simulink model "Kaltitude"  (R2015a)
settings: Solver=ode2  StartTime=0.0  StopTime=10.0  FixedStep=0.01  RelTol=1e-3
InitFcn:
  | Parameters
settings Model: Creator=pela  LastModifiedBy=Mattia
settings HardwareCC: ProdLargestAtomicInteger=Long  ProdLargestAtomicFloat=Double  ProdEndianess=LittleEndian  ProdHWDeviceType=ARM Compatible->ARM Cortex
settings RTWCC: GenCodeOnly=on  GenerateReport=on  Toolchain=Microsoft Visual C++ 2013 v12.0 | nmake (64-bit Windows)  BuildConfiguration=Faster Runs  LaunchReport=on  TargetLang=C++
settings GRTTargetCC: MatFileLogging=off  MultiInstanceERTCode=on  CodeInterfacePackaging=C++ class  SupportNonFinite=off

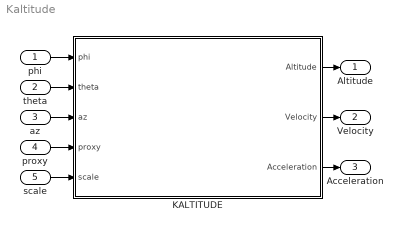
== system Kaltitude ==
  phi : Inport
  theta : Inport  Port=2
  az : Inport  Port=3
  proxy : Inport  Port=4
  scale : Inport  Port=5
  KALTITUDE : Subsystem
  Altitude : Outport
  Velocity : Outport  Port=2
  Acceleration : Outport  Port=3
  wires:
  phi/1 -> KALTITUDE/1(phi)
  theta/1 -> KALTITUDE/2(theta)
  az/1 -> KALTITUDE/3(az)
  proxy/1 -> KALTITUDE/4(proxy)
  KALTITUDE/1(Altitude) -> Altitude/1
  KALTITUDE/2(Velocity) -> Velocity/1
  KALTITUDE/3(Acceleration) -> Acceleration/1
  scale/1 -> KALTITUDE/5(scale)

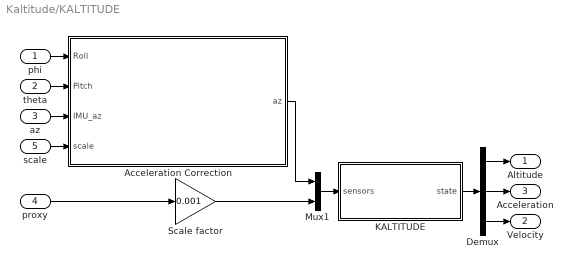
== system Kaltitude/KALTITUDE ==
  phi : Inport
  theta : Inport  Port=2
  az : Inport  Port=3
  proxy : Inport  Port=4
  scale : Inport  Port=5
  Acceleration Correction : MATLAB Function  TreatAsAtomicUnit=on
  Demux : Demux  Outputs=3
  KALTITUDE : Subsystem
  Mux1 : Mux  Inputs=2
  Scale factor : Gain  Gain=0.001
  Altitude : Outport
  Velocity : Outport  Port=2
  Acceleration : Outport  Port=3
  wires:
  az/1 -> Acceleration Correction/3(IMU_az)
  phi/1 -> Acceleration Correction/1(Roll)
  theta/1 -> Acceleration Correction/2(Pitch)
  Mux1/1 -> KALTITUDE/1(sensors)
  proxy/1 -> Scale factor/1
  Scale factor/1 -> Mux1/2
  Acceleration Correction/1(az) -> Mux1/1
  KALTITUDE/1(state) -> Demux/1
  Demux/1 -> Altitude/1
  Demux/2 -> Acceleration/1
  Demux/3 -> Velocity/1
  scale/1 -> Acceleration Correction/4(scale)

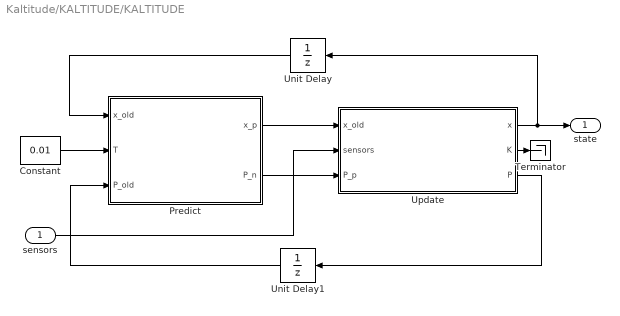
== system Kaltitude/KALTITUDE/KALTITUDE ==
  sensors : Inport
  Constant : Constant  Value=0.01  VectorParams1D=off  SampleTime=-1
  "Predict " : MATLAB Function  TreatAsAtomicUnit=on
  Terminator : Terminator
  Unit Delay : UnitDelay  InitialCondition=zeros(3,1)  SampleTime=-1
  Unit Delay1 : UnitDelay  InitialCondition=eye(3)*0.001  SampleTime=-1
  Update : MATLAB Function  TreatAsAtomicUnit=on
  state : Outport
  wires:
  Update/2(K) -> Terminator/1
  Unit Delay1/1 -> "Predict "/3(P_old)
  Update/1(x) -> state/1, Unit Delay/1
  "Predict "/1(x_p) -> Update/1(x_old)
  sensors/1 -> Update/2(sensors)
  "Predict "/2(P_n) -> Update/3(P_p)
  Constant/1 -> "Predict "/2(T)
  Update/3(P) -> Unit Delay1/1
  Unit Delay/1 -> "Predict "/1(x_old)

== matlab function Kaltitude/KALTITUDE/Acceleration Correction ==
  data: Roll input; Pitch input; IMU_az input; scale input; az output
function az = Accelerometer_correction(Roll,Pitch,IMU_az,scale)
%#codegen
acc_norm = IMU_az/scale;
a_corr = sqrt(1 - (sin(Roll)^2 + sin(Pitch)^2));

az = (acc_norm - a_corr)*9.81;

== matlab function Kaltitude/KALTITUDE/KALTITUDE/Update ==
  data x_old settings: description=A-priori state estimate.
  data sensors settings: description=Measurements from the sensors.
  data x settings: description=Corrected state estimate.
  data P_p settings: description=A-priori covariance estimate.
  data P settings: description=Corrected covariance estimate.
  data: x_old input; sensors input; x output; K output; P_p input; P output
%%A-KF state correction   %
% Author: Matteo Ferronato%
% Last review: 2016/02/09 %
%%%%%%%%%%%%%%%%%%%%%%%%%%%
function [x,K,P] = state_update(x_old,sensors,P_p)
% Useful Parameters
Rn = [0.7  0 ;
       0   1];
%%
H = [0 1 0 ;
     1 0 0];

%%
h = H*x_old;

%%
Pl = P_p;
x_p = x_old;

for j = 1:2
    % Innovation covariance
    S = H(j,:)*Pl*H(j,:)' + Rn(j,j);
    
    % Kalman gain
    K = Pl*H(j,:)'/S;
    
    % Updated state estimate
    x_p = x_p + K*(sensors(j,1)-h(j,1));
    
    % Updated estimated covariance
    Pl = (eye(3) - K*H(j,:))*Pl*(eye(3) - K*H(j,:))' + K*Rn(j,j)*K';
end

P = Pl;
x = x_p;

== matlab function Kaltitude/KALTITUDE/KALTITUDE/Predict  ==
  data x_old settings: description=State estimate at the previous step.
  data x_p settings: description=A-priori state estimate.
  data T settings: description=Control signal at the previous step.
  data P_n settings: description=A-priori covariance estimate.
  data P_old settings: description=Covariance estimate at the previous step.
  data: x_old input; x_p output; T input; P_n output; P_old input
%%AKF state update        %
% Author: Matteo Ferronato%
% Last review: 2016/02/09 %
%%%%%%%%%%%%%%%%%%%%%%%%%%%
function [x_p,P_n] = state_predict(x_old,T,P_old)
%% State-noise matrix
Qn = [0.005   0     0   ;
        0   0.005   0   ;
        0     0   0.005];

%% Dynamics matrix
A = [ 1, T^2/2, T;
      0,   1,   0;
      0,   T,   1];

x_p = A*x_old;

%% Covariance propagation
P_n = A*P_old*A' + Qn;
